simulink model "SynthFSE"  (R2024a)
settings: Solver=ode45  StartTime=0.0  StopTime=1780  RelTol=1e-3  EnableMultiTasking=on
undefined symbols (not defined in the file or in its folder): j, QAM
libraries: hdlBasic x71, dspmlti4 x2, hdlUtilities x1, vmcUtilities x1
(part 2 of 2)

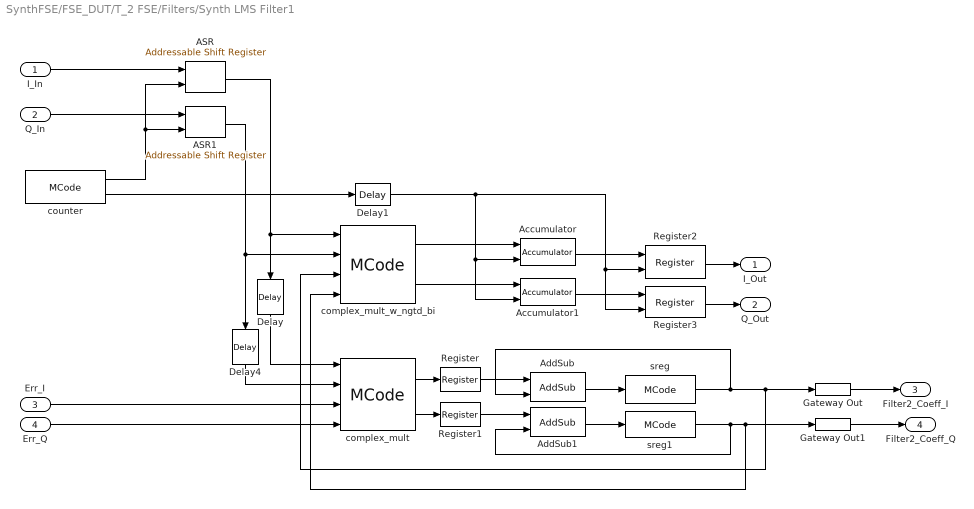
== system SynthFSE/FSE_DUT/T_2 FSE/Filters/Synth LMS Filter1 ==
  I_In : Inport
  Q_In : Inport  Port=2
  Err_I : Inport  Port=3
  Err_Q : Inport  Port=4
  ASR : hdlBasic/Addressable Shift Register  infer_latency=off  depth=4  initVector=[0]  en=off  use_behavioral_HDL=on  Optimization=Resource  use_rpm=on  XmcBlockStatus=1  maskContainerNames=group1  block_type=addrsr  block_config=sysgen:Addrsr_config
  ASR1 : hdlBasic/Addressable Shift Register  infer_latency=off  depth=4  initVector=[0]  en=off  use_behavioral_HDL=on  Optimization=Resource  use_rpm=on  XmcBlockStatus=1  maskContainerNames=group1  block_type=addrsr  block_config=sysgen:Addrsr_config
  Accumulator : hdlBasic/Accumulator  operation=Add  n_bits=36  overflow=Wrap  scale=1  rst=on  hasbypass=off  en=off  latency=1  msb_inp=100  msb=100  lsb=-100  use_behavioral_HDL=on  implementation=Fabric  XmcBlockStatus=1  maskContainerNames=group3  block_type=accum  block_config=sysgen:Accum_config  block_width=566  block_height=845
  Accumulator1 : hdlBasic/Accumulator  operation=Add  n_bits=36  overflow=Wrap  scale=1  rst=on  hasbypass=off  en=off  latency=1  msb_inp=100  msb=100  lsb=-100  use_behavioral_HDL=on  implementation=Fabric  XmcBlockStatus=1  maskContainerNames=group3  block_type=accum  block_config=sysgen:Accum_config  block_width=566  block_height=845
  AddSub : hdlBasic/AddSub  mode=Addition  use_carryin=off  use_carryout=off  en=off  latency=0  precision=User Defined  arith_type="Signed  (2's comp)"  n_bits=18  bin_pt=10  quantization="Round  (unbiased: +/- Inf)"  overflow=Saturate  use_behavioral_HDL=on  hw_selection=Fabric  pipelined=off  use_rpm=on  XmcBlockStatus=1  maskContainerNames=tabcontainer1  block_type=addsub  block_config=sysgen:Addsub_config
  AddSub1 : hdlBasic/AddSub  mode=Addition  use_carryin=off  use_carryout=off  en=off  latency=0  precision=User Defined  arith_type="Signed  (2's comp)"  n_bits=18  bin_pt=10  quantization="Round  (unbiased: +/- Inf)"  overflow=Saturate  use_behavioral_HDL=on  hw_selection=Fabric  pipelined=off  use_rpm=on  XmcBlockStatus=1  maskContainerNames=tabcontainer1  block_type=addsub  block_config=sysgen:Addsub_config
  Delay : hdlBasic/Delay  rst=off  en=off  latency=27  reg_retiming=off  XmcBlockStatus=1  maskContainerNames=group1  block_type=delay  block_config=sysgen:Delay_config
  Delay1 : hdlBasic/Delay  rst=off  en=off  latency=3  reg_retiming=on  XmcBlockStatus=1  maskContainerNames=group1  block_type=delay  block_config=sysgen:Delay_config
  Delay4 : hdlBasic/Delay  rst=off  en=off  latency=27  reg_retiming=off  XmcBlockStatus=1  maskContainerNames=group1  block_type=delay  block_config=sysgen:Delay_config
  Gateway Out : hdlBasic/Gateway Out  inherit_from_input=off  bool_to_boolean=off  hdl_port=off  rows=1  columns=1  UseAsDAC=off  DACChannel='1'  interface=None  automatic_assignment=on  address_offset=hex2dec('00')  intf_name=''  intf_description=''  timing_constraint=None  locs_specified=off  LOCs={}  io_standard={}  XmcBlockStatus=1  maskContainerNames=group4  block_type=gatewayout  block_config=sysgen:gateway_out_config  block_width_w=590  block_height_w=620  block_width=620  block_height=750
  Gateway Out1 : hdlBasic/Gateway Out  inherit_from_input=off  bool_to_boolean=off  hdl_port=off  rows=1  columns=1  UseAsDAC=off  DACChannel='1'  interface=None  automatic_assignment=on  address_offset=hex2dec('00')  intf_name=''  intf_description=''  timing_constraint=None  locs_specified=off  LOCs={}  io_standard={}  XmcBlockStatus=1  maskContainerNames=group4  block_type=gatewayout  block_config=sysgen:gateway_out_config  block_width_w=590  block_height_w=620  block_width=620  block_height=750
  Register : hdlBasic/Register  init=0  rst=off  en=off  XmcBlockStatus=1  maskContainerNames=tabcontainer1  block_type=register  block_config=sysgen:Register_config
  Register1 : hdlBasic/Register  init=0  rst=off  en=off  XmcBlockStatus=1  maskContainerNames=tabcontainer1  block_type=register  block_config=sysgen:Register_config
  Register2 : hdlBasic/Register  init=0  rst=off  en=on  XmcBlockStatus=1  maskContainerNames=tabcontainer1  block_type=register  block_config=sysgen:Register_config
  Register3 : hdlBasic/Register  init=0  rst=off  en=on  XmcBlockStatus=1  maskContainerNames=tabcontainer1  block_type=register  block_config=sysgen:Register_config
  complex_mult : hdlBasic/MCode  mfname=complex_mult  explicit_period=off  period=1  iptable={'ar','';'ai','';'br','';'bi','';'negate_bi',' 0'}  optable={'pr','off';'pi','off'}  enable_stdout=off  enable_debug=off  suppress_output=off  defparams={'negate_bi', 0}  hide_port_list={}  block_type=mcode  block_width=444  block_height=788
      settings: infoedit=Pass input values to a MATLAB function for evaluation in Xilinx fixed-point type. The input ports of the block are input arguments of the function. The output ports of the block are output arguments of the function.  block_version=8.1
  complex_mult_w_ngtd_bi : hdlBasic/MCode  mfname=complex_mult  explicit_period=off  period=1  iptable={'ar','';'ai','';'br','';'bi','';'negate_bi',' 1'}  optable={'pr','off';'pi','off'}  enable_stdout=off  enable_debug=off  suppress_output=off  defparams={'negate_bi', 1}  hide_port_list={}  block_type=mcode  block_width=444  block_height=788
      settings: infoedit=Pass input values to a MATLAB function for evaluation in Xilinx fixed-point type. The input ports of the block are input arguments of the function. The output ports of the block are output arguments of the function.  block_version=8.1
  counter : hdlBasic/MCode  mfname=fir_fsm  explicit_period=on  period=1  iptable={'reset',' false';'init',' 3'}  optable={'cnt','off';'rst','off'}  enable_stdout=off  enable_debug=off  suppress_output=off  defparams={'reset', false,'init', 3}  hide_port_list={}  block_type=mcode  block_width=444  block_height=788
      settings: infoedit=Pass input values to a MATLAB function for evaluation in Xilinx fixed-point type. The input ports of the block are input arguments of the function. The output ports of the block are output arguments of the function.  block_version=8.1
  sreg : hdlBasic/MCode  mfname=sreg  explicit_period=off  period=1  iptable={'din','';'len','4';'init','init_i'}  optable={'q','off'}  enable_stdout=off  enable_debug=off  suppress_output=off  defparams={'len',4,'init',init_i}  hide_port_list={}  block_type=mcode  block_width=444  block_height=788
      settings: infoedit=Pass input values to a MATLAB function for evaluation in Xilinx fixed-point type. The input ports of the block are input arguments of the function. The output ports of the block are output arguments of the function.  block_version=8.1
  sreg1 : hdlBasic/MCode  mfname=sreg  explicit_period=off  period=1  iptable={'din','';'len','4';'init','init_q'}  optable={'q','off'}  enable_stdout=off  enable_debug=off  suppress_output=off  defparams={'len',4,'init',init_q}  hide_port_list={}  block_type=mcode  block_width=444  block_height=788
      settings: infoedit=Pass input values to a MATLAB function for evaluation in Xilinx fixed-point type. The input ports of the block are input arguments of the function. The output ports of the block are output arguments of the function.  block_version=8.1
  I_Out : Outport  VectorParamsAs1DForOutWhenUnconnected=off
  Q_Out : Outport  Port=2  VectorParamsAs1DForOutWhenUnconnected=off
  Filter2_Coeff_I : Outport  Port=3  VectorParamsAs1DForOutWhenUnconnected=off
  Filter2_Coeff_Q : Outport  Port=4  VectorParamsAs1DForOutWhenUnconnected=off
  wires:
  sreg1/1 -> AddSub1/2, Gateway Out1/1, complex_mult_w_ngtd_bi/4
  Delay4/1 -> complex_mult/2
  Delay/1 -> complex_mult/1
  Accumulator/1 -> Register2/1
  Delay1/1 -> Accumulator1/2, Accumulator/2, Register2/2, Register3/2
  complex_mult_w_ngtd_bi/1 -> Accumulator/1
  complex_mult_w_ngtd_bi/2 -> Accumulator1/1
  Accumulator1/1 -> Register3/1
  Register1/1 -> AddSub1/1
  Register/1 -> AddSub/1
  sreg/1 -> AddSub/2, Gateway Out/1, complex_mult_w_ngtd_bi/3
  counter/2 -> Delay1/1
  counter/1 -> ASR1/2, ASR/2
  AddSub1/1 -> sreg1/1
  AddSub/1 -> sreg/1
  Gateway Out1/1 -> Filter2_Coeff_Q/1
  Gateway Out/1 -> Filter2_Coeff_I/1
  Err_I/1 -> complex_mult/3
  Err_Q/1 -> complex_mult/4
  complex_mult/2 -> Register1/1
  complex_mult/1 -> Register/1
  Register2/1 -> I_Out/1
  Register3/1 -> Q_Out/1
  ASR/1 -> Delay/1, complex_mult_w_ngtd_bi/1
  ASR1/1 -> Delay4/1, complex_mult_w_ngtd_bi/2
  I_In/1 -> ASR/1
  Q_In/1 -> ASR1/1
